simulink model "PR_Pick_and_Place"  (R2023b)
settings: Solver=FixedStepAuto  StartTime=0.0  StopTime=Te  FixedStep=Ts  RelTol=1e-3  EnableMultiTasking=on
values from neighbouring files (symbols this model uses):
  rEend = [0.25; 0.04; 0]    [PR_init_PnP.m]
  rEstart = [0.25; 0.25; 0]    [PR_init_PnP.m]
settings Model: Creator=Hoebarth  LastModifiedBy=Flo
settings SolverCC: AlgebraicLoopSolver=TrustRegion
settings DataIOCC: LimitDataPoints=on  SaveFormat=Array  SignalLoggingSaveFormat=ModelDataLogs  ReturnWorkspaceOutputs=off
settings OptimizationCC: LifeSpan=inf
settings DebuggingCC: SaveWithParameterizedLinksMsg=none  UnderspecifiedInitializationDetection=Classic  MergeDetectMultiDrivingBlocksExec=none  SignalResolutionControl=TryResolveAllWithWarning  MultiTaskDSMMsg=warning  MultiTaskCondExecSysMsg=none  UnconnectedInputMsg=warning  UnconnectedOutputMsg=warning  UnconnectedLineMsg=warning  SFUnexpectedBacktrackingDiag=warning  SFNoUnconditionalDefaultTransitionDiag=warning  SFExecutionAtInitializationDiag=none  ArithmeticOperatorsInVariantConditions=warning
settings HardwareCC: ProdBitPerPointer=32  ProdBitPerSizeT=32  ProdBitPerPtrDiffT=32  ProdLargestAtomicFloat=None  ProdIntDivRoundTo=Undefined  ProdEndianess=Unspecified  ProdWordSize=32  ProdHWDeviceType=32-bit Generic  TargetUnknown=on
settings ModelReferenceCC: EnableRefExpFcnMdlSchedulingChecks=on  PropagateSignalLabelsOutOfModel=off
settings SFSimCC: SimUseLocalCustomCode=off  SimParseCustomCode=off  CustomCodeUndefinedFunction=UseInterfaceOnly
settings RTWCC: RTWUseLocalCustomCode=off
settings CodeAppCC: StateflowObjectComments=on
settings GRTTargetCC: TargetFcnLib=ansi_tfl_tmw.mat  TargetLangStandard=C89/C90 (ANSI)  CombineOutputUpdateFcns=off  GRTInterface=on
settings ConfigComp: CovMetricSettings=dw  CovSaveCumulativeToWorkspaceVar=on  CovSaveSingleToWorkspaceVar=on  CovExternalEMLEnable=off

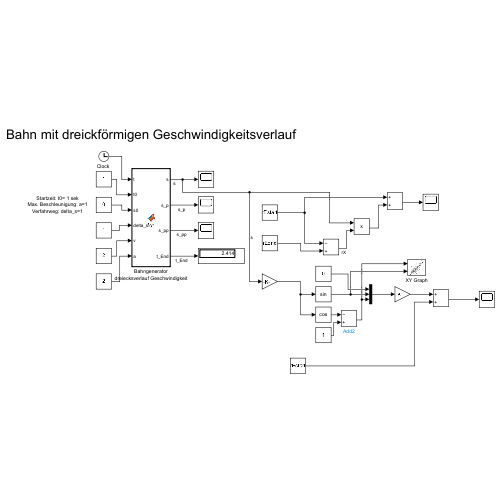
[thumbnail: Simulink's stored preview of the top-level diagram]
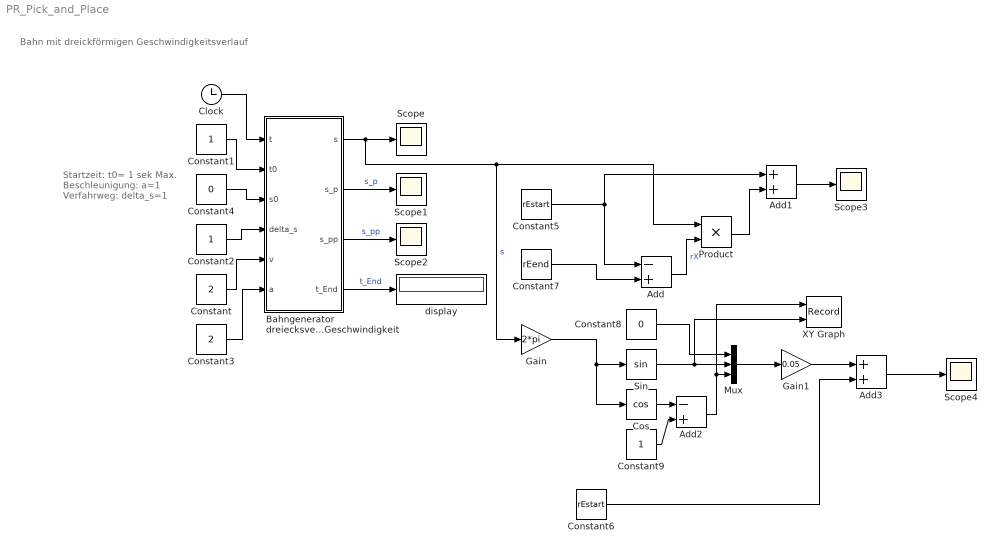
== system PR_Pick_and_Place ==
  note: Bahn mit dreickförmigen Geschwindigkeitsverlauf
  note: Startzeit: t0= 1 sek
      | Max. Beschleunigung: a=1
      | Verfahrweg: delta_s=1
  Add : Sum  Inputs=-+
  Add1 : Sum
  Add2 : Sum  Inputs=-+
  Add3 : Sum
  Bahngenerator dreiecksverlauf Geschwindigkeit : MATLAB Function  TreatAsAtomicUnit=on
  "Clock " : Clock
  Constant : Constant  Value=2
  Constant1 : Constant
  Constant2 : Constant
  Constant3 : Constant  Value=2
  Constant4 : Constant  Value=0
  Constant5 : Constant  Value=rEstart
  Constant6 : Constant  Value=rEstart
  Constant7 : Constant  Value=rEend
  Constant8 : Constant  Value=0
  Constant9 : Constant
  Cos : Trigonometry  Operator=cos
  Gain : Gain  Gain=2*pi
  Gain1 : Gain  Gain=0.05
  Mux : Mux  Inputs=3
  Product : Product
  Scope{,1..4} (5 alike) : Scope
  Sin : Trigonometry
  XY Graph : Record  FileSettingsInternal="{\"entries\":[{\"content\":{\"excelSettings\":{\"content\":{},\"type\":\"Streamout.ExcelSettings\"}},\"type\":\"Streamout.FileSettingStorage\",\"uuid\":\"\"}],\"packageUris\":[\"http:\\/\\/schema.mathworks.com\\/mf0\\/streamout_blocks\\/R2020a\"],\"version\":\"1.0\"}"  Layout=[1 1]  SignalsInternal="{\"entries\":[{\"content\":{\"signals\":[{\"content\":{\"blockPath\":[],\"dimensions\":[1],\"domain\":\"\",\"lineColor\":\"#a2142f\",\"plots\":[1],\"port\":1,\"sid\":[\"\"],\"signalID\":37,\"signalName\":\"Add2\"},\"type\":\"RecordBlkView.Signal\",\"uuid\":\"\"},{\"content\":{\"blockPath\":[],\"dimensions\":[1],\"domain\":\"\",\"lineColor\":\"#139fff\",\"plots\":[1],\"port\":2,\"sid\":[\"\"],\"signalID\":41,\"signalName\":\"Sin\"},\"type\":\"RecordBlkView.Signal\",\"uuid\":\"\"}]},\"type\":\"RecordBlkView.InputSignals\",\"uuid\":\"\"}],\"packageUris\":[\"http:\\/\\/schema.mathworks.com\\/mf0\\/streamout_blocks\\/R2020a\"],\"version\":\"1.0\"}"  VisualizationBindings="{\"xyplotplugin\":{\"info\":[{\"series\":[{\"bindingParametersList\":[{\"parameter\":\"X-Axis\",\"signalID\":37,\"signalName\":\"Add2\"},{\"parameter\":\"Y-Axis\",\"signalID\":41,\"signalName\":\"Sin\"}],\"seriesID\":64451}],\"subplotID\":1}]}}"  CompatibilityTag=XY
  display : Display
  wires:
  "Clock "/1 -> Bahngenerator dreiecksverlauf Geschwindigkeit/1(t)
  Constant1/1 -> Bahngenerator dreiecksverlauf Geschwindigkeit/2(t0)
  Constant4/1 -> Bahngenerator dreiecksverlauf Geschwindigkeit/3(s0)
  Bahngenerator dreiecksverlauf Geschwindigkeit/4(t_End) -> display/1  "t_End"
  Bahngenerator dreiecksverlauf Geschwindigkeit/2(s_p) -> Scope1/1  "s_p"
  Bahngenerator dreiecksverlauf Geschwindigkeit/3(s_pp) -> Scope2/1  "s_pp"
  Constant2/1 -> Bahngenerator dreiecksverlauf Geschwindigkeit/4(delta_s)
  Constant3/1 -> Bahngenerator dreiecksverlauf Geschwindigkeit/6(a)
  Constant/1 -> Bahngenerator dreiecksverlauf Geschwindigkeit/5(v)
  Constant5/1 -> Add/1, Add1/1
  Constant7/1 -> Add/2
  Add/1 -> Product/2  "rX"
  Product/1 -> Add1/2
  Add1/1 -> Scope3/1
  Bahngenerator dreiecksverlauf Geschwindigkeit/1(s) -> Gain/1, Product/1, Scope/1  "s"
  Add3/1 -> Scope4/1
  Constant6/1 -> Add3/2
  Gain/1 -> Sin/1, Cos/1
  Constant8/1 -> Mux/1
  Sin/1 -> XY Graph/2, Mux/2
  Mux/1 -> Gain1/1
  Gain1/1 -> Add3/1
  Cos/1 -> Add2/1
  Add2/1 -> XY Graph/1, Mux/3
  Constant9/1 -> Add2/2

== matlab function PR_Pick_and_Place/Bahngenerator dreiecksverlauf Geschwindigkeit ==
  data: t input; s output; t0 input; s0 input; delta_s input; v input; a input; s_p output; s_pp output; t_End output
function [s, s_p, s_pp, t_End] = fcn(t, t0, s0, delta_s, v, a)
%#codegen

% Mein erster Bahngenerator:
% in embeded Matlab functions kann mit gewoehnlichem m-Code (Matlab Code)
% gearbeitet werden.

% todo: Implementierung Bahngenerator

tb = v / a;
tfrei = (-v*tb + abs(delta_s))/v;
Ta = 2 * sqrt(abs(delta_s)/a);
if tfrei > 0
    if t < t0
        s = 0;
        s_p = 0;
        s_pp = 0;
    elseif t < t0 + tb
        s = a/2 * (-t0 + t)^2;
        s_p = a * (t - t0);
        s_pp = a;
    elseif t < t0 + tb + tfrei
        s = a/2 * tb * (2*t - tb - 2*t0);
        s_p = a * (tb);
        s_pp = 0;
    elseif t < t0 + 2*tb + tfrei
        s = a*(-tb^2 + (2*t - 2*t0 -tfrei)*tb - (-t0 - tfrei +t)^2 /2);
        s_p = a * (t0 + 2*tb +tfrei - t);
        s_pp = -a;
    else
        s = a*tb*(tb +tfrei);
        s_p = 0;
        s_pp = 0;
    end
    t_End = t0 + 2*tb + tfrei;
else
    if t < t0
        s = 0;
        s_p = 0;
        s_pp = 0;
    elseif t < t0 + Ta/2
        s = a/2 * (-t0 + t)^2;
        s_p = a * (t - t0);
        s_pp = a;
    elseif t < t0 + Ta
        s = a/2 * (-Ta^2 / 2 + 2*(t - t0)*Ta - (t - t0)^2);
        s_p = a * (t0 + Ta - t);
        s_pp = -a;
    else
        s = a*Ta^2/4;
        s_p = 0;
        s_pp = 0;
    end
   
    t_End = t0 + Ta;
end
s = s * sign(delta_s) + s0;
s_p = s_p * sign(delta_s);
s_pp = s_pp * sign(delta_s);
